simulink model "problem_2_sim"  (R2025a)
settings: Solver=VariableStepAuto  StartTime=0.0  StopTime=t_sim  RelTol=1e-3
values from neighbouring files (symbols this model uses):
  C = [1 0]    [problem_2.m]
  Kq = K(1)    [problem_2.m]
  Kx = K(2:3)    [problem_2.m]
  Ts = 0.05    [problem_2.m]
undefined symbols (not defined in the file or in its folder): DiscIntNeverNeededParam
libraries: cstblocks x1
settings Model: Creator=s360159  LastModifiedBy=s360159

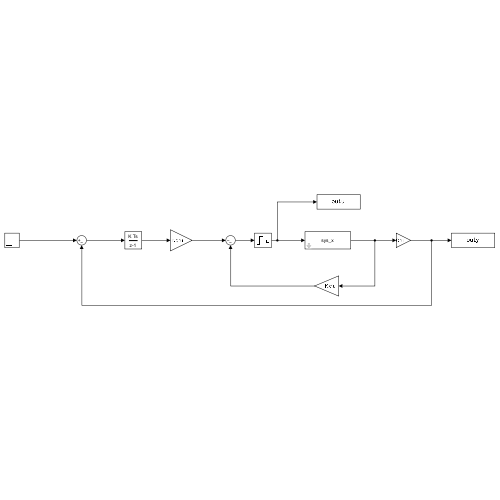
[thumbnail: Simulink's stored preview of the top-level diagram]
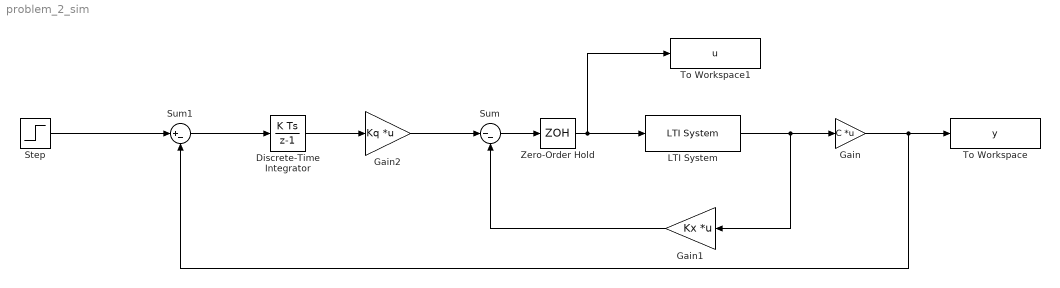
== system problem_2_sim ==
  Discrete-Time Integrator : DiscreteIntegrator  SampleTime=Ts  ICPrevOutput=DiscIntNeverNeededParam  ICPrevScaledInput=DiscIntNeverNeededParam
  Gain : Gain  Gain=C  Multiplication=Matrix(K*u)
  Gain1 : Gain  Gain=Kx  Multiplication=Matrix(K*u)
  Gain2 : Gain  Gain=Kq  Multiplication=Matrix(K*u)
  LTI System : cstblocks/LTI System  sys=sys_x  IC=x0  PadeOrder=0
  Step : Step  Time=0  SampleTime=Ts
  Sum : Sum  Inputs=|--
  Sum1 : Sum  Inputs=|+-
  To Workspace : ToWorkspace  VariableName=y  SaveFormat=Timeseries  SampleTime=Ts
  To Workspace1 : ToWorkspace  VariableName=u  SaveFormat=Timeseries  SampleTime=Ts
  Zero-Order Hold : ZeroOrderHold  SampleTime=Ts
  wires:
  LTI System/1 -> Gain1/1, Gain/1
  Gain/1 -> Sum1/2, To Workspace/1
  Zero-Order Hold/1 -> To Workspace1/1, LTI System/1
  Gain1/1 -> Sum/2
  Gain2/1 -> Sum/1
  Sum/1 -> Zero-Order Hold/1
  Discrete-Time Integrator/1 -> Gain2/1
  Sum1/1 -> Discrete-Time Integrator/1
  Step/1 -> Sum1/1
